simulink model "HILSimulation"  (R2024b)
settings: Solver=FixedStepAuto  StartTime=0.0  StopTime=inf  RelTol=1e-3
model workspace (MAT data in the model file):
  NumRxValues = 4
  NumTxVariables = 1
undefined symbols (not defined in the file or in its folder): f
libraries: instrumentlib x2
settings Model: Creator=natha  LastModifiedBy=natha

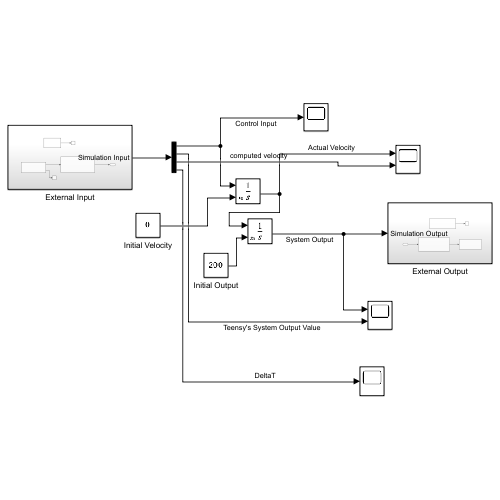
[thumbnail: Simulink's stored preview of the top-level diagram]
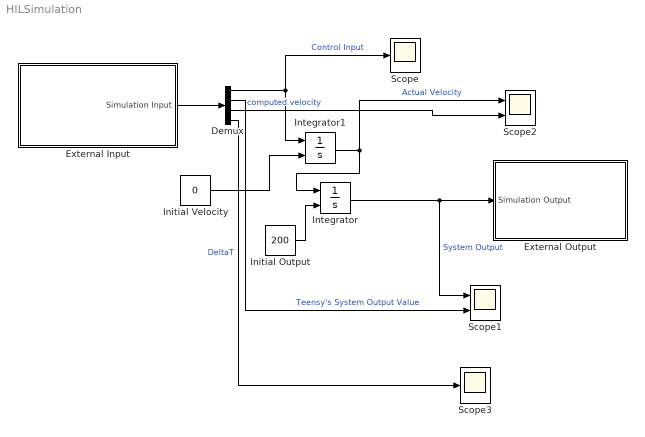
== system HILSimulation ==
  Demux : Demux  Outputs=NumRxValues
  External Input : Subsystem
  External Output : Subsystem
  Initial Output : Constant  Value=200
  Initial Velocity : Constant  Value=0
  Integrator : Integrator  InitialConditionSource=external
  Integrator1 : Integrator  InitialConditionSource=external
  Scope : Scope
  Scope1 : Scope  NumInputPorts=2
  Scope2 : Scope  NumInputPorts=2
  Scope3 : Scope
  wires:
  Integrator/1 -> External Output/1(Simulation Output), Scope1/1  "System Output"
  Initial Output/1 -> Integrator/2
  Demux/1 -> Integrator1/1, Scope/1  "Control Input"
  External Input/1(Simulation Input) -> Demux/1
  Demux/2 -> Scope1/2  "Teensy's System Output Value"
  Integrator1/1 -> Scope2/1, Integrator/1  "Actual Velocity"
  Initial Velocity/1 -> Integrator1/2
  Demux/3 -> Scope2/2  "computed velocity"
  Demux/4 -> Scope3/1  "DeltaT"

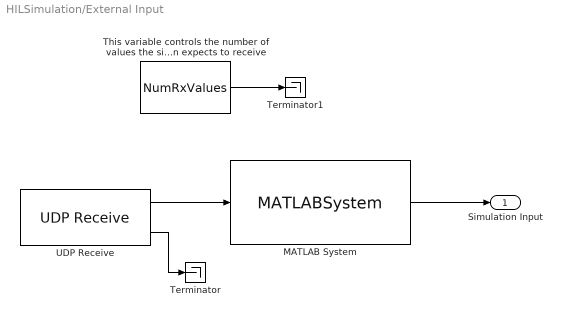
== system HILSimulation/External Input ==
  MATLAB System : MATLABSystem  System=BytesToFloats  NumValues=NumRxValues  SimulateUsing=Code generation
      mask Type: BytesToFloats
      mask Display:
      | disp('BytesToFloats');
      | port_label('input',1,'bytes');
      | port_label('output',1,'floatValues');
  Terminator : Terminator
  Terminator1 : Terminator
  This variable controls the number of values the simulation expects to receive : Constant  Value=NumRxValues
  UDP Receive : instrumentlib/UDP Receive  LocalAddress=127.0.0.1  LocalPort=25000  EnablePortSharing=off  Host=localhost  Port=25001  GetLatestData=on  DataSize=[ 1, 8*NumRxValues ]  DataType=uint8  ASCIIFormatting=%f,  Terminator=LF  CustomTerminator=10  ByteOrder=big-endian  EnableBlockingMode=off  Timeout=10  SampleTime=0.01  SimulateUsing=Interpreted execution
  Simulation Input : Outport
  wires:
  UDP Receive/1 -> MATLAB System/1
  MATLAB System/1 -> Simulation Input/1
  UDP Receive/2 -> Terminator/1
  This variable controls the number of values the simulation expects to receive/1 -> Terminator1/1

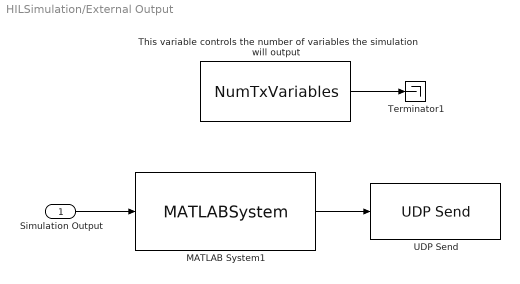
== system HILSimulation/External Output ==
  Simulation Output : Inport
  MATLAB System1 : MATLABSystem  System=FloatsToBytes  NumValues=NumTxVariables  SimulateUsing=Code generation
      mask Type: FloatsToBytes
      mask Display:
      | disp('FloatsToBytes');
      | port_label('input',1,'floatValues');
      | port_label('output',1,'bytes');
  Terminator1 : Terminator
  This variable controls the number of variables the simulation will output : Constant  Value=NumTxVariables
  UDP Send : instrumentlib/UDP Send  Host=127.0.0.1  Port=25001  LocalAddress=127.0.0.1  LocalPort=25000  EnablePortSharing=off  OutputDatagramPacketSize=8 * NumTxVariables  ByteOrder=big-endian  EnableBlockingMode=off  SimulateUsing=Interpreted execution
  wires:
  MATLAB System1/1 -> UDP Send/1
  Simulation Output/1 -> MATLAB System1/1
  This variable controls the number of variables the simulation will output/1 -> Terminator1/1
